simulink model "passivity_based_control_project"  (R2024b)
settings: Solver=VariableStepAuto  StartTime=0.0  StopTime=tot_time  RelTol=1e-3
values from neighbouring files (symbols this model uses):
  Do = 50*eye(3)    [passivity_based_control.m]
  g = 9.81    [main.m]    (also in mpc_control.m)
  Ib = diag([1.2416, 1.2416, 2 * 1.2416])    [getQuadrotorDynamicsAndJacobian.m]    (also in linearized_model.m = diag([Ib1 Ib2 Ib3]); main.m = diag([1.2416 1.2416 2*1.2416]))
  Kd = diag([100 10 100])    [passivity_based_control.m]
  Ko = sigma*Do    [passivity_based_control.m]
  Kp = 50*lqr(A, B, Q_p, R_p)    [hierarchical_control.m]    (also in passivity_based_control.m = diag([100 20 100]))
  lin_vel_0 = [0 0 0]    [planner_1.m]    (also in planner_2.m = dot_p_d(1:3,1)')
  mass = 1.2    [getQuadrotorDynamicsAndJacobian.m]    (also in main.m)
  ni = 5    [passivity_based_control.m]
  pos_0 = waypoints(1,1:3)    [planner_1.m]    (also in planner_2.m = p_d(1:3,1)')
  sigma = 10    [passivity_based_control.m]
  Ts = 0.001    [main.m]
  u_T0 = 11.772    [main.m]
  w_bb_0 = [0 0 0]    [planner_1.m]    (also in planner_2.m)
undefined symbols (not defined in the file or in its folder): dspblkCoreblockFVToolHelper, gcbh
libraries: robotcorelib x1, uavutilslib x1
settings Model: Creator=fabioruggiero  LastModifiedBy=marcomaffeo
settings ModelReferenceCC: EnableRefExpFcnMdlSchedulingChecks=on
settings RTWCC: GPUComputeCapability=3.5

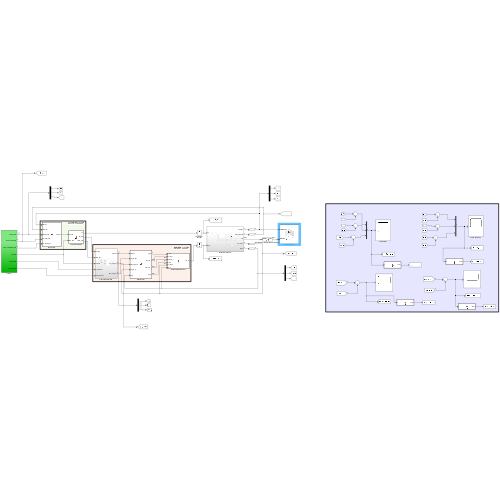
[thumbnail: Simulink's stored preview of the top-level diagram]
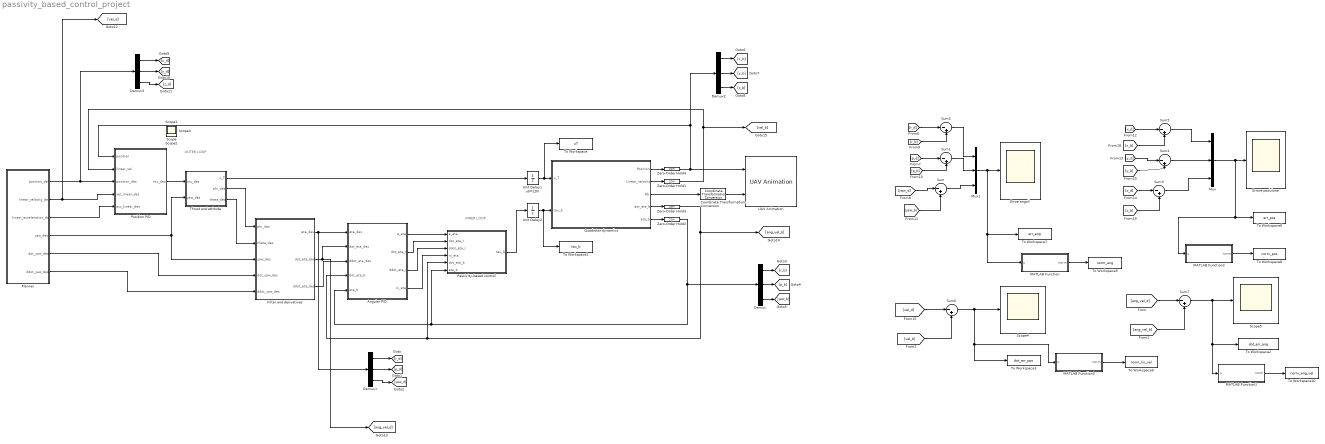
== system passivity_based_control_project ==
  note: INNER LOOP
  note: OUTER LOOP
  Angular PID : MATLAB Function  TreatAsAtomicUnit=on
  Coordinate Transformation Conversion : robotcorelib/Coordinate Transformation Conversion  InputRepresentation=Rotation Matrix  InputEulerSequence=ZYX  ShowTrVecInputPort=on  OutputRepresentation=Quaternion  OutputEulerSequence=ZYX  ShowTrVecOutputPort=on  SimulateUsing=Interpreted execution
  Demux{,1..3} (4 alike) : Demux  Outputs=3
  Erroe angoli : Scope
  Errore posizione : Scope
  Filter and derivatives : Subsystem
  MATLAB Function : MATLAB Function  TreatAsAtomicUnit=on
  MATLAB Function1 : MATLAB Function  TreatAsAtomicUnit=on
  MATLAB Function2 : MATLAB Function  TreatAsAtomicUnit=on
  MATLAB Function3 : MATLAB Function  TreatAsAtomicUnit=on
  Mux : Mux  Inputs=3
  Mux1 : Mux  Inputs=3
  Passivity-based control : MATLAB Function  TreatAsAtomicUnit=on
  Planner : Subsystem
  Position PID : MATLAB Function  TreatAsAtomicUnit=on
  Quadrotor dynamics : Subsystem
  Scope{,1..5} (6 alike) : Scope
  Sum{,1..7} (8 alike) : Sum  Inputs=|-+
  Thrust and attitude : MATLAB Function  TreatAsAtomicUnit=on
  To Workspace : ToWorkspace  VariableName=uT  SaveFormat=Structure With Time  SampleTime=-1
  To Workspace1 : ToWorkspace  VariableName=tau_b  SaveFormat=Structure With Time  SampleTime=-1
  To Workspace10 : ToWorkspace  VariableName=norm_ang_vel  SaveFormat=Structure With Time  SampleTime=-1
  To Workspace2 : ToWorkspace  VariableName=dot_err_ang  SaveFormat=Structure With Time  SampleTime=-1
  To Workspace3 : ToWorkspace  VariableName=dot_err_pos  SaveFormat=Structure With Time  SampleTime=-1
  To Workspace5 : ToWorkspace  VariableName=norm_ang  SaveFormat=Structure With Time  SampleTime=-1
  To Workspace6 : ToWorkspace  VariableName=err_pos  SaveFormat=Structure With Time  SampleTime=-1
  To Workspace7 : ToWorkspace  VariableName=err_ang  SaveFormat=Structure With Time  SampleTime=-1
  To Workspace8 : ToWorkspace  VariableName=norm_pos  SaveFormat=Structure With Time  SampleTime=-1
  To Workspace9 : ToWorkspace  VariableName=norm_lin_vel  SaveFormat=Structure With Time  SampleTime=-1
  UAV Animation : uavutilslib/UAV Animation  NumUAV=1  DynamicUAVConfig=off  UAVType=Multirotor  UAVSize=1  UAVColor=[0 0 1]  UAVTrajectoryAlpha=1  InertialZDirection=Down  RotationFormat=Quaternion  DrawMarkers=off  SampleTime=0.01
  Unit Delay1 u0=12N : UnitDelay  InitialCondition=u_T0  SampleTime=Ts
  Unit Delay2 : UnitDelay  SampleTime=Ts
  Zero-Order Hold{1..4} (4 alike) : ZeroOrderHold  SampleTime=Ts
  wires:
  Position PID/1(mu_des) -> Thrust and attitude/1(mu_des)
  Unit Delay1 u0=12N/1 -> To Workspace/1, Quadrotor dynamics/1(u_T)
  Quadrotor dynamics/1(Position) -> Zero-Order Hold4/1
  Quadrotor dynamics/2(Linear_velocity) -> Zero-Order Hold1/1
  Planner/1(position_des) -> Position PID/3(position_des), Demux3/1
  Planner/2(linear_velocity_des) -> [vel_d], Position PID/4(vel_linear_des)
  Quadrotor dynamics/5(eta_b) -> Zero-Order Hold2/1
  Coordinate Transformation Conversion/1 -> UAV Animation/2
  Planner/3(linear_acceleration_des) -> Position PID/5(acc_linear_des)
  Planner/4(yaw_des) -> Thrust and attitude/2(yaw_des), Filter and derivatives/3(yaw_des)
  Thrust and attitude/1(u_T) -> Unit Delay1 u0=12N/1
  Planner/5(dot_yaw_des) -> Filter and derivatives/4(dot_yaw_des)
  Planner/6(ddot_yaw_des) -> Filter and derivatives/5(ddot_yaw_des)
  Filter and derivatives/2(dot_eta_des) -> [ang_vel_d], Angular PID/2(dot_eta_des)
  Filter and derivatives/3(ddot_eta_des) -> Angular PID/3(ddot_eta_des)
  Passivity-based control/1(tau_b) -> Unit Delay2/1
  Quadrotor dynamics/4(dot_eta_b) -> Zero-Order Hold3/1
  Zero-Order Hold4/1 -> Demux2/1, Position PID/1(position), UAV Animation/1
  Quadrotor dynamics/3(Rb) -> Coordinate Transformation Conversion/1
  Filter and derivatives/1(eta_des) -> Angular PID/1(eta_des), Demux1/1
  Demux1/1 -> [r_d]
  Demux1/2 -> [p_d]
  Demux1/3 -> [yaw_d]
  Thrust and attitude/2(phi_des) -> Filter and derivatives/1(phi_des)
  Thrust and attitude/3(theta_des) -> Filter and derivatives/2(theta_des)
  Demux/1 -> [r_b]
  Demux/2 -> [p_b]
  Demux/3 -> [yaw_b]
  Demux2/3 -> [z_b]
  Demux2/1 -> [x_b]
  Demux2/2 -> [y_b]
  Demux3/2 -> [y_d]
  Demux3/3 -> [z_d]
  Demux3/1 -> [x_d]
  Angular PID/2(dot_eta_r) -> Passivity-based control/2(dot_eta_r)
  Angular PID/3(ddot_eta_r) -> Passivity-based control/3(ddot_eta_r)
  Angular PID/1(e_eta) -> Passivity-based control/1(e_eta)
  Angular PID/4(ni_eta) -> Passivity-based control/4(ni_eta)
  Zero-Order Hold1/1 -> [vel_b], Position PID/2(linear_vel)
  Zero-Order Hold2/1 -> Demux/1, Passivity-based control/6(eta_b), Angular PID/5(eta_b)
  Zero-Order Hold3/1 -> [ang_vel_b], Angular PID/4(dot_eta_b), Passivity-based control/5(dot_eta_b)
  Unit Delay2/1 -> To Workspace1/1, Quadrotor dynamics/2(tau_b)
  [p_b] -> Sum1/2
  Sum7/1 -> Scope5/1, MATLAB Function1/1(u), To Workspace2/1
  [p_d] -> Sum1/1
  [x_d] -> Sum5/1
  [r_b] -> Sum2/2
  [ang_vel_b] -> Sum7/2
  MATLAB Function/1(norm) -> To Workspace5/1
  [yaw_b] -> Sum/2
  MATLAB Function2/1(norm) -> To Workspace8/1
  Sum2/1 -> Mux1/1
  [vel_b] -> Sum6/2
  MATLAB Function3/1(norm) -> To Workspace9/1
  Mux/1 -> MATLAB Function2/1(u), To Workspace6/1, Errore posizione/1
  Sum5/1 -> Mux/1
  Sum/1 -> Mux1/3
  Sum1/1 -> Mux1/2
  [y_b] -> Sum4/2
  Sum6/1 -> Scope4/1, MATLAB Function3/1(u), To Workspace3/1
  [yaw_d] -> Sum/1
  [ang_vel_d] -> Sum7/1
  Mux1/1 -> Erroe angoli/1, To Workspace7/1, MATLAB Function/1(u)
  [z_d] -> Sum3/1
  [y_d] -> Sum4/1
  [x_b] -> Sum5/2
  MATLAB Function1/1(norm) -> To Workspace10/1
  [z_b] -> Sum3/2
  Sum3/1 -> Mux/3
  Sum4/1 -> Mux/2
  [r_d] -> Sum2/1
  [vel_d] -> Sum6/1

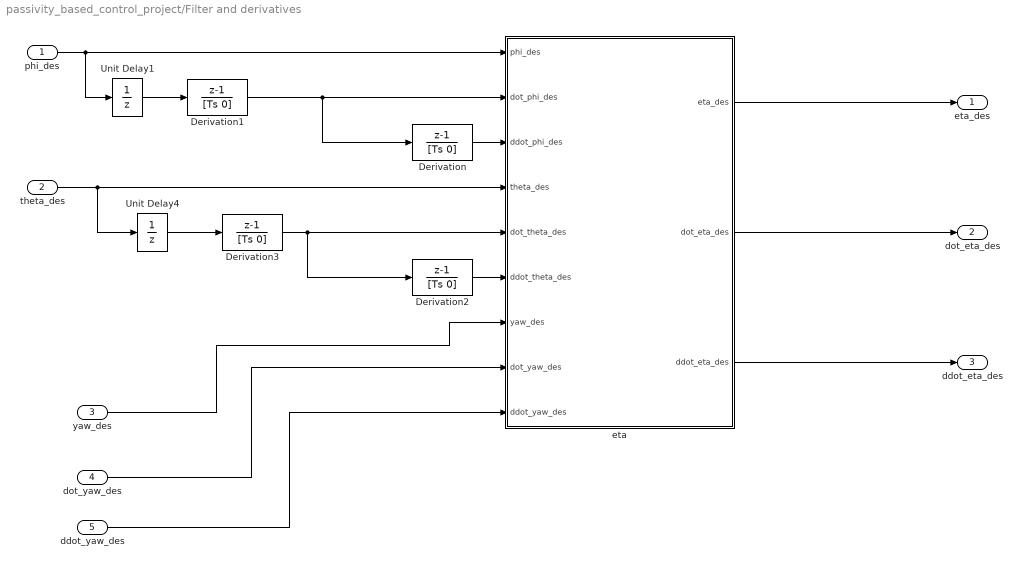
== system passivity_based_control_project/Filter and derivatives ==
  phi_des : Inport
  theta_des : Inport  Port=2
  yaw_des : Inport  Port=3
  dot_yaw_des : Inport  Port=4
  ddot_yaw_des : Inport  Port=5
  Derivation{,1..3} (4 alike) : DiscreteTransferFcn  LoadFcn=dspblkCoreblockFVToolHelper(gcbh,'load');  Numerator=[1 -1]  Denominator=[Ts 0]  SampleTime=Ts
      settings: CopyFcn=dspblkCoreblockFVToolHelper(gcbh,'copy');  DeleteFcn=dspblkCoreblockFVToolHelper(gcbh,'close');  ModelCloseFcn=dspblkCoreblockFVToolHelper(gcbh,'close');  PreSaveFcn=dspblkCoreblockFVToolHelper(gcbh,'presave');  PostSaveFcn=dspblkCoreblockFVToolHelper(gcbh,'postsave');  CloseFcn=dspblkCoreblockFVToolHelper(gcbh,'close');
  Unit Delay1 : UnitDelay  SampleTime=Ts
  Unit Delay4 : UnitDelay  SampleTime=Ts
  eta : MATLAB Function  TreatAsAtomicUnit=on
  eta_des : Outport
  dot_eta_des : Outport  Port=2
  ddot_eta_des : Outport  Port=3
  wires:
  yaw_des/1 -> eta/7(yaw_des)
  dot_yaw_des/1 -> eta/8(dot_yaw_des)
  ddot_yaw_des/1 -> eta/9(ddot_yaw_des)
  eta/1(eta_des) -> eta_des/1
  phi_des/1 -> eta/1(phi_des), Unit Delay1/1
  Derivation/1 -> eta/3(ddot_phi_des)
  Derivation2/1 -> eta/6(ddot_theta_des)
  theta_des/1 -> Unit Delay4/1, eta/4(theta_des)
  eta/2(dot_eta_des) -> dot_eta_des/1
  eta/3(ddot_eta_des) -> ddot_eta_des/1
  Unit Delay4/1 -> Derivation3/1
  Unit Delay1/1 -> Derivation1/1
  Derivation1/1 -> Derivation/1, eta/2(dot_phi_des)
  Derivation3/1 -> Derivation2/1, eta/5(dot_theta_des)

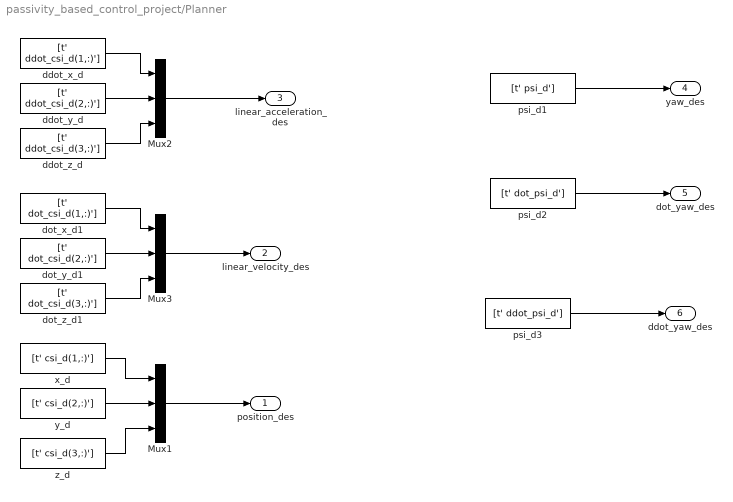
== system passivity_based_control_project/Planner ==
  Mux1 : Mux  Inputs=3
  Mux2 : Mux  Inputs=3
  Mux3 : Mux  Inputs=3
  ddot_x_d : FromWorkspace  VariableName=[t' ddot_csi_d(1,:)']  SampleTime=Ts
  ddot_y_d : FromWorkspace  VariableName=[t' ddot_csi_d(2,:)']  SampleTime=Ts
  ddot_z_d : FromWorkspace  VariableName=[t' ddot_csi_d(3,:)']  SampleTime=Ts
  dot_x_d1 : FromWorkspace  VariableName=[t' dot_csi_d(1,:)']  SampleTime=Ts
  dot_y_d1 : FromWorkspace  VariableName=[t' dot_csi_d(2,:)']  SampleTime=Ts
  dot_z_d1 : FromWorkspace  VariableName=[t' dot_csi_d(3,:)']  SampleTime=Ts
  psi_d1 : FromWorkspace  VariableName=[t' psi_d']  SampleTime=Ts
  psi_d2 : FromWorkspace  VariableName=[t' dot_psi_d']  SampleTime=Ts
  psi_d3 : FromWorkspace  VariableName=[t' ddot_psi_d']  SampleTime=Ts
  x_d : FromWorkspace  VariableName=[t' csi_d(1,:)']  SampleTime=Ts
  y_d : FromWorkspace  VariableName=[t' csi_d(2,:)']  SampleTime=Ts
  z_d : FromWorkspace  VariableName=[t' csi_d(3,:)']  SampleTime=Ts
  position_des : Outport
  linear_velocity_des : Outport  Port=2
  linear_acceleration_des : Outport  Port=3
  yaw_des : Outport  Port=4
  dot_yaw_des : Outport  Port=5
  ddot_yaw_des : Outport  Port=6
  wires:
  z_d/1 -> Mux1/3
  y_d/1 -> Mux1/2
  dot_z_d1/1 -> Mux3/3
  Mux1/1 -> position_des/1
  Mux3/1 -> linear_velocity_des/1
  ddot_z_d/1 -> Mux2/3
  ddot_x_d/1 -> Mux2/1
  dot_y_d1/1 -> Mux3/2
  x_d/1 -> Mux1/1
  dot_x_d1/1 -> Mux3/1
  ddot_y_d/1 -> Mux2/2
  Mux2/1 -> linear_acceleration_des/1
  psi_d1/1 -> yaw_des/1
  psi_d2/1 -> dot_yaw_des/1
  psi_d3/1 -> ddot_yaw_des/1

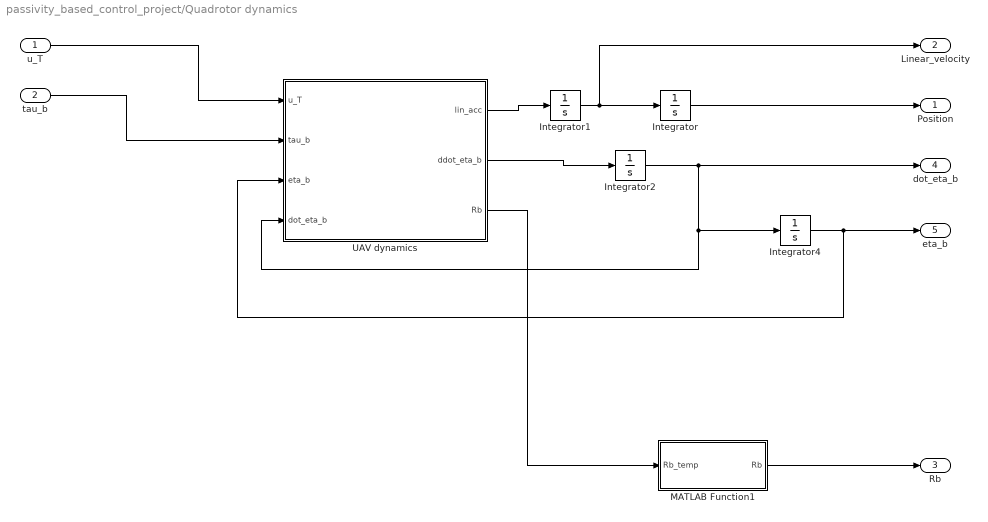
== system passivity_based_control_project/Quadrotor dynamics ==
  u_T : Inport
  tau_b : Inport  Port=2
  Integrator : Integrator  InitialCondition=pos_0
  Integrator1 : Integrator  InitialCondition=lin_vel_0
  Integrator2 : Integrator  InitialCondition=[0 0 0]
  Integrator4 : Integrator  InitialCondition=w_bb_0
  MATLAB Function1 : MATLAB Function  TreatAsAtomicUnit=on
  UAV dynamics : MATLAB Function  TreatAsAtomicUnit=on
  Position : Outport
  Linear_velocity : Outport  Port=2
  Rb : Outport  Port=3
  dot_eta_b : Outport  Port=4
  eta_b : Outport  Port=5
  wires:
  tau_b/1 -> UAV dynamics/2(tau_b)
  Integrator/1 -> Position/1
  UAV dynamics/1(lin_acc) -> Integrator1/1
  u_T/1 -> UAV dynamics/1(u_T)
  Integrator1/1 -> Linear_velocity/1, Integrator/1
  Integrator2/1 -> UAV dynamics/4(dot_eta_b), Integrator4/1, dot_eta_b/1
  Integrator4/1 -> UAV dynamics/3(eta_b), eta_b/1
  MATLAB Function1/1(Rb) -> Rb/1
  UAV dynamics/2(ddot_eta_b) -> Integrator2/1
  UAV dynamics/3(Rb) -> MATLAB Function1/1(Rb_temp)

== matlab function passivity_based_control_project/Angular PID ==
  data: eta_des input size=3; e_eta output size=3; dot_eta_des input size=3; ddot_eta_des input size=3; dot_eta_b input size=3; eta_b input size=3; dot_eta_r output; ddot_eta_r output; ni_eta output; sigma parameter; ni parameter
function [e_eta,dot_eta_r,ddot_eta_r,ni_eta] = fcn(eta_des,dot_eta_des,ddot_eta_des,dot_eta_b,eta_b, sigma, ni)

%tracking error for the attitude

e_eta = eta_b-eta_des;
dot_e_eta = dot_eta_b-dot_eta_des;

dot_eta_r=dot_eta_des-sigma*e_eta;
ddot_eta_r=ddot_eta_des-ni*dot_e_eta;

ni_eta=dot_e_eta+sigma*e_eta;



end

== matlab function passivity_based_control_project/Passivity-based control ==
  data: e_eta input; dot_eta_r input; ddot_eta_r input size=3; ni_eta input; dot_eta_b input size=3; tau_b output size=3; eta_b input size=3; Ib parameter; Do parameter; Ko parameter
function tau_b = fcn(e_eta,dot_eta_r,ddot_eta_r,ni_eta,dot_eta_b,eta_b, Ib, Do, Ko)

%matrix def
Q=[1              0                         -sin(eta_b(2));
   0        cos(eta_b(1))  cos(eta_b(2))*sin(eta_b(1));
   0       -sin(eta_b(1))  cos(eta_b(1))*cos(eta_b(2))];

Q_dot=[0   0                                                                                                -cos(eta_b(2))*dot_eta_b(2);
           0 -sin(eta_b(1))*dot_eta_b(1) -sin(eta_b(2))*sin(eta_b(1))*dot_eta_b(2)+cos(eta_b(2))*cos(eta_b(1))*dot_eta_b(1);
           0 -cos(eta_b(1))*dot_eta_b(1) -sin(eta_b(2))*cos(eta_b(1))*dot_eta_b(2)-cos(eta_b(2))*sin(eta_b(1))*dot_eta_b(1)];

S = skew(Q*(dot_eta_b));
C = Q'*S*Ib*Q + Q'*Ib*Q_dot; 

M=Q'*Ib*Q;


tau_b = (inv(Q)')*((M*ddot_eta_r)+(C*dot_eta_r)-(Do*ni_eta)-Ko*e_eta);


end

function S = skew(v)
if(numel(v)~= 1)
S= [0 -v(3) v(2); 
    v(3) 0 -v(1);
    -v(2) v(1) 0];
else
S= zeros(3);
end
end

== matlab function passivity_based_control_project/MATLAB Function ==
  data: u input; norm output
function norm = fcn(u)

norm = sqrt(u(1)^2+u(2)^2+u(3)^2);

== matlab function passivity_based_control_project/MATLAB Function1 ==
  data: u input; norm output
function norm = fcn(u)

norm = sqrt(u(1)^2+u(2)^2+u(3)^2);

== matlab function passivity_based_control_project/MATLAB Function2 ==
  data: u input; norm output
function norm = fcn(u)

norm = sqrt(u(1)^2+u(2)^2+u(3)^2);

== matlab function passivity_based_control_project/MATLAB Function3 ==
  data: u input; norm output
function norm = fcn(u)

norm = sqrt(u(1)^2+u(2)^2+u(3)^2);

== matlab function passivity_based_control_project/Thrust and attitude ==
  data: mu_des input size=3; u_T output size=1; yaw_des input size=1; phi_des output size=1; theta_des output size=1; g parameter; mass parameter
function [u_T,phi_des,theta_des] = fcn(mu_des,yaw_des, g, mass)

eps=1e-2;

%flat outputs

u_T = mass*sqrt((mu_des(1)^2)+(mu_des(2)^2)+((mu_des(3)-g)^2));

phi_des = asin((mass/u_T)* ((mu_des(2)*cos(yaw_des))-(mu_des(1)*sin(yaw_des))));

den = mu_des(3) - g;

if abs(den) < eps
    den = sign(den)*eps;
end
theta_des = atan((mu_des(1)*cos(yaw_des)+(mu_des(2)*sin(yaw_des)))/den);
end

== matlab function passivity_based_control_project/Quadrotor dynamics/UAV dynamics ==
  data: u_T input size=1; tau_b input size=3; lin_acc output size=3; ddot_eta_b output size=3; eta_b input size=3; dot_eta_b input size=3; Rb output size=[3,3]; Ib parameter; mass parameter
function [lin_acc, ddot_eta_b,Rb] = fcn(u_T,tau_b,eta_b,dot_eta_b, Ib, mass)

%matrix definition
Q=[1              0                        -sin(eta_b(2));
   0        cos(eta_b(1))     cos(eta_b(2))*sin(eta_b(1));
   0       -sin(eta_b(1))    cos(eta_b(1))*cos(eta_b(2))];

Q_dot=[0             0                                                                          -cos(eta_b(2))*dot_eta_b(2);
       0 -sin(eta_b(1))*dot_eta_b(1)     -sin(eta_b(2))*sin(eta_b(1))*dot_eta_b(2)+cos(eta_b(2))*cos(eta_b(1))*dot_eta_b(1);
       0 -cos(eta_b(1))*dot_eta_b(1)     -sin(eta_b(2))*cos(eta_b(1))*dot_eta_b(2)-cos(eta_b(2))*sin(eta_b(1))*dot_eta_b(1)];


M=Q'*Ib*Q;

S = skew(Q*(dot_eta_b));

C = (Q'*S*Ib*Q)+ (Q'*Ib*Q_dot); 


Rb=[cos(eta_b(2))*cos(eta_b(3))   sin(eta_b(1))*sin(eta_b(2))*cos(eta_b(3))-cos(eta_b(1))*sin(eta_b(3))   cos(eta_b(1))*sin(eta_b(2))*cos(eta_b(3))+sin(eta_b(1))*sin(eta_b(3));
    cos(eta_b(2))*sin(eta_b(3))   sin(eta_b(1))*sin(eta_b(2))*sin(eta_b(3))+cos(eta_b(1))*cos(eta_b(3))   cos(eta_b(1))*sin(eta_b(2))*sin(eta_b(3))-sin(eta_b(1))*cos(eta_b(3));
        -sin(eta_b(2))              sin(eta_b(1))*cos(eta_b(2))                                           cos(eta_b(1))*cos(eta_b(2))];


%quadcopter dynamic model
lin_acc = 9.81*[0 0 1]'-(u_T/mass)*Rb*[0 0 1]';

ddot_eta_b = (inv(M))*((-C*dot_eta_b)+(Q'*tau_b));


end

function S = skew(v)
if(numel(v)~= 1)
S= [0 -v(3) v(2); 
    v(3) 0 -v(1);
    -v(2) v(1) 0];
else
S= zeros(3);
end
end

== matlab function passivity_based_control_project/Position PID ==
  data: position input size=3; mu_des output size=3; linear_vel input size=3; position_des input size=3; vel_linear_des input size=3; acc_linear_des input size=3; Kp parameter; Kd parameter
function mu_des  = fcn(position, linear_vel,...
position_des, vel_linear_des, acc_linear_des, Kp, Kd)

%tracking errors for the translational motion
err_p = position - position_des;
dot_err_p = linear_vel - vel_linear_des;


%virtual desired accelteration

mu_des= (-Kd*dot_err_p)-(Kp*err_p) + acc_linear_des;

== matlab function passivity_based_control_project/Filter and derivatives/eta ==
  data: eta_des output size=3; phi_des input size=1; dot_phi_des input size=1; ddot_phi_des input size=1; theta_des input size=1; dot_theta_des input size=1; ddot_theta_des input size=1; yaw_des input size=1; dot_yaw_des input size=1; ddot_yaw_des input size=1; dot_eta_des output size=3; ddot_eta_des output size=3
function [eta_des,dot_eta_des,ddot_eta_des] = fcn(phi_des,dot_phi_des, ddot_phi_des, theta_des, dot_theta_des, ...
    ddot_theta_des, yaw_des,dot_yaw_des,ddot_yaw_des)

%desired attitude,velocity and acceleration


eta_des = [phi_des; theta_des; yaw_des];

dot_eta_des = [dot_phi_des; dot_theta_des; dot_yaw_des];

ddot_eta_des = [ddot_phi_des; ddot_theta_des; ddot_yaw_des];

end

== matlab function passivity_based_control_project/Quadrotor dynamics/MATLAB Function1 ==
  data: Rb_temp input; Rb output
function Rb = fcn(Rb_temp)
    [U,S,V] = svd(Rb_temp);
    sigma = det(U*V');
    S_ = diag([1 1 sigma]);

    Rb = U*S_*V';
end
